simulink model "aero_atc"  (Simulink 6.0)
settings: Solver=ode45  StartTime=0.0  StopTime=60000  MaxStep=.25  RelTol=1e-3
PreLoadFcn:
  | aero_preload_atc
InitFcn:
  | aero_init_atc
values from neighbouring files (symbols this model uses):
  AZ_Sep = get(findobj('Tag','AZ_Sep_edit'),'Value')    [aero_init_atc.m]
  BwPw = get(findobj('Tag','BW_PW_edit'),'Value')    [aero_init_atc.m]
  E = get(findobj('Tag','Antenna_E_edit'),'Value')    [aero_init_atc.m]
  EL_Sep = get(findobj('Tag','EL_Sep_edit'),'Value')    [aero_init_atc.m]
  Lambda = get(findobj('Tag','Wavelength_edit'),'Value')    [aero_init_atc.m]
  Loss = get(findobj('Tag','Losses_edit'),'Value')    [aero_init_atc.m]
  Noise = get(findobj('Tag','Noise_Factor_edit'),'Value')    [aero_init_atc.m]
  Pt = get(findobj('Tag','Trans_Power_edit'),'Value')    [aero_init_atc.m]
  rainfall = get(findobj('Style','radiobutton','Value',[1]),'UserData')    [aero_init_atc.m]
  Rrange = get(findobj('Tag','RADAR_Range_edit'),'Value')    [aero_init_atc.m]
  Rres = get(findobj('Tag','Range_Res_edit'),'Value')    [aero_init_atc.m]
  SNR = get(findobj('Tag','SNR_edit'),'Value')    [aero_init_atc.m]
  Temp = get(findobj('Tag','Working_Temp_edit'),'Value')    [aero_init_atc.m]
libraries: simulink3 x1
CloseFcn:
  | aero_atcscript('close')
settings Model: RequirementInfo=9  CovMetricSettings=d  Creator=The MathWorks Inc.  LastModifiedBy=batserve  ExtModeTrigMode=oneshot  ExtModeArmWhenConnect=off  ExtModeAutoUpdateStatusClock=off
settings DataIOCC: MaxDataPoints=5000  SaveOutput=off  SaveTime=off
settings OptimizationCC: BlockReduction=off  BooleanDataType=off
settings DebuggingCC: CheckExecutionContextPreStartOutputMsg=on  CheckExecutionContextRuntimeOutputMsg=on  SolverPrmCheckMsg=none
settings HardwareCC: TargetUnknown=on

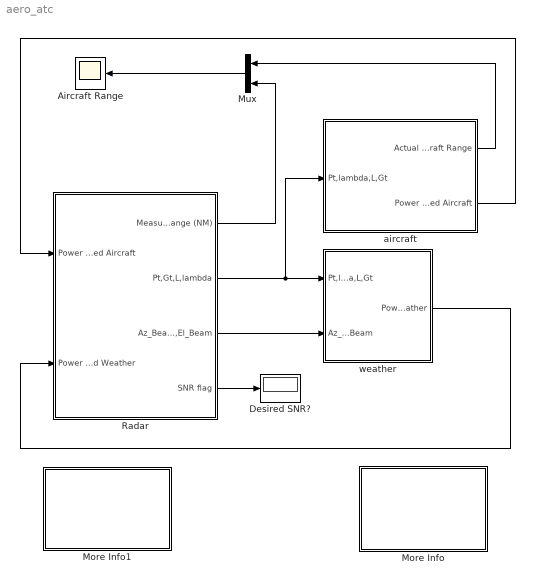
== system aero_atc ==
  Aircraft Range : Scope
      settings: DeleteFcn=simscope BlockIsBeingDestroyed  TimeRange=10300  YMin=0  YMax=65
  Desired SNR? : Display
  More Info : Subsystem  PropExecContextAcrossSSBoundary=on
      settings: OpenFcn=aero_atcscript
      mask Display: disp('Double-click \nhere for \ninformation on \nthis demonstration')
  More Info1 : Subsystem  PropExecContextAcrossSSBoundary=on
      settings: OpenFcn=simcad(bdroot);
      mask Display: disp('Double click\nhere for\nSimulink Help')
  Mux : Mux  Orientation=left  Inputs=2
  Radar : Subsystem  PropExecContextAcrossSSBoundary=on
      mask Display: image(radar)
  aircraft : Subsystem  PropExecContextAcrossSSBoundary=on
      mask Display: image(plane)
  weather : Subsystem  PropExecContextAcrossSSBoundary=on
      mask Display: image(weather);
  wires:
  Radar/2(Pt,Gt,L,lambda) -> aircraft/1(Pt,lambda,L,Gt), weather/1(Pt,lambda,L,Gt)
  Radar/3(Az_Beam,El_Beam) -> weather/2(Az_Beam,El_Beam)
  weather/1(Power Returned Weather) -> Radar/2(Power Received Weather)
  aircraft/2(Power Returned Aircraft) -> Radar/1(Power Received Aircraft)
  Radar/1(Measured Aircraft Range (NM)) -> Mux/2
  aircraft/1(Actual Aircraft Range) -> Mux/1
  Mux/1 -> Aircraft Range/1
  Radar/4(SNR flag) -> Desired SNR?/1

== system aero_atc/More Info ==

== system aero_atc/More Info1 ==

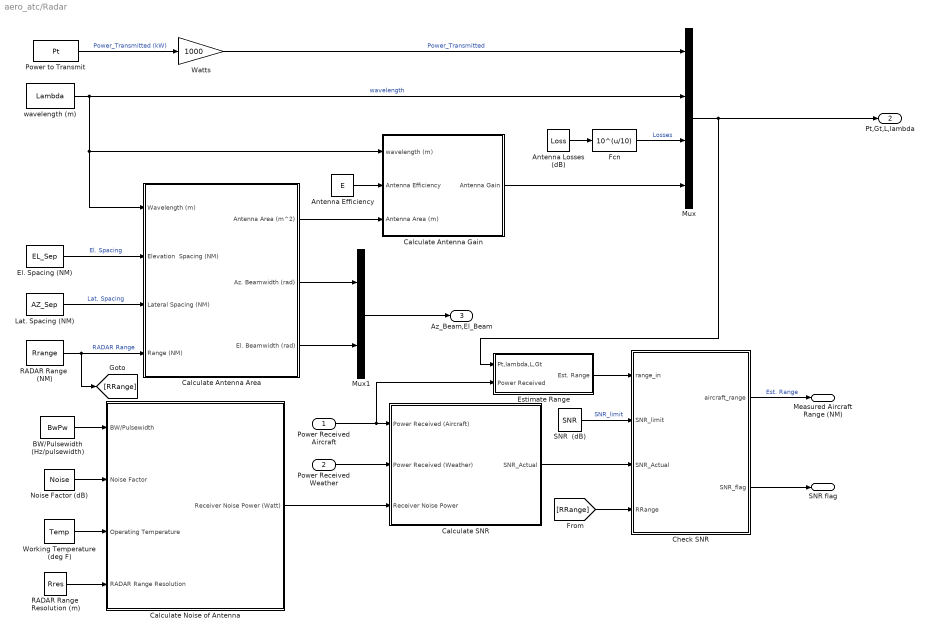
== system aero_atc/Radar ==
  Power Received Aircraft : Inport  Port=1  LatchInput=off
  Power Received Weather : Inport  Port=2  LatchInput=off
  Antenna Efficiency : Constant  Value=E
  Antenna Losses (dB) : Constant  Value=Loss
  BW/Pulsewidth (Hz/pulsewidth) : Constant  Value=BwPw
  Calculate SNR : Subsystem  PropExecContextAcrossSSBoundary=on
  Calculate Antenna Area : Subsystem  PropExecContextAcrossSSBoundary=on
  Calculate Antenna Gain : Subsystem  PropExecContextAcrossSSBoundary=on
  Calculate Noise of Antenna : Subsystem  PropExecContextAcrossSSBoundary=on
  Check SNR : Stateflow chart  PropExecContextAcrossSSBoundary=on
  El. Spacing (NM) : Constant  Value=EL_Sep
  Estimate Range : Subsystem  PropExecContextAcrossSSBoundary=on
  Fcn : Fcn  Expr=10^(u/10)
  Lat. Spacing (NM) : Constant  Value=AZ_Sep
  Mux : Mux
  Mux1 : Mux  Inputs=2
  Noise Factor (dB) : Constant  Value=Noise
  Power to Transmit : Constant  Value=Pt
  RADAR Range  (NM) : Constant  Value=Rrange
  RADAR Range  Resolution (m) : Constant  Value=Rres
  SNR  (dB) : Constant  Value=SNR
  Watts : Gain  Gain=1000  SaturateOnIntegerOverflow=on
  Working Temperature (deg F) : Constant  Value=Temp
  "wavelength (m) " : Constant  Value=Lambda
  Measured Aircraft Range (NM) : Outport
  Pt,Gt,L,lambda : Outport  Port=2
  Az_Beam,El_Beam : Outport  Port=3
  SNR flag : Outport  Port=4
  wires:
  Antenna Efficiency/1 -> Calculate Antenna Gain/2(Antenna Efficiency)
  Lat. Spacing (NM)/1 -> Calculate Antenna Area/3(Lateral Spacing (NM))  "Lat. Spacing"
  El. Spacing (NM)/1 -> Calculate Antenna Area/2(Elevation  Spacing (NM))  "El. Spacing"
  "wavelength (m) "/1 -> Calculate Antenna Area/1(Wavelength (m)), Calculate Antenna Gain/1(wavelength (m)), Mux/2  "wavelength"
  Calculate Antenna Area/1(Antenna Area (m^2)) -> Calculate Antenna Gain/3(Antenna Area (m))
  RADAR Range  (NM)/1 -> Calculate Antenna Area/4(Range (NM)), [RRange]  "RADAR Range"
  RADAR Range  Resolution (m)/1 -> Calculate Noise of Antenna/4(RADAR Range Resolution)
  BW/Pulsewidth (Hz/pulsewidth)/1 -> Calculate Noise of Antenna/1(BW/Pulsewidth)
  Noise Factor (dB)/1 -> Calculate Noise of Antenna/2(Noise Factor)
  Working Temperature (deg F)/1 -> Calculate Noise of Antenna/3(Operating Temperature)
  Calculate Antenna Area/3("El. Beamwidth (rad) ") -> Mux1/2
  Calculate Antenna Area/2("Az. Beamwidth (rad) ") -> Mux1/1
  Mux1/1 -> Az_Beam,El_Beam/1
  Power Received Weather/1 -> Calculate SNR/2(Power Received (Weather))
  Power Received Aircraft/1 -> Calculate SNR/1(Power Received (Aircraft)), Estimate Range/2(Power Received)
  Calculate Noise of Antenna/1(Receiver Noise Power (Watt)) -> Calculate SNR/3(Receiver Noise Power)
  Mux/1 -> Pt,Gt,L,lambda/1, Estimate Range/1(Pt,lambda,L,Gt)
  Calculate Antenna Gain/1("Antenna Gain ") -> Mux/4
  Fcn/1 -> Mux/3  "Losses"
  Watts/1 -> Mux/1  "Power_Transmitted"
  Antenna Losses (dB)/1 -> Fcn/1
  Power to Transmit/1 -> Watts/1  "Power_Transmitted (kW)"
  Check SNR/1(aircraft_range) -> Measured Aircraft Range (NM)/1  "Est. Range"
  Estimate Range/1(Est. Range) -> Check SNR/1(range_in)
  SNR  (dB)/1 -> Check SNR/2(SNR_limit)  "SNR_limit"
  Calculate SNR/1(SNR_Actual) -> Check SNR/3(SNR_Actual)
  [RRange] -> Check SNR/4(RRange)
  Check SNR/2(SNR_flag) -> SNR flag/1

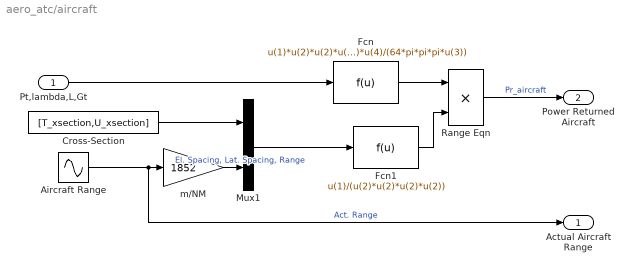
== system aero_atc/aircraft ==
  Pt,lambda,L,Gt : Inport  Port=1  LatchInput=off
  Aircraft Range : Sin  Amplitude=25  Bias=35  Frequency=0.0025  SampleTime=0
  Cross-Section : FromWorkspace  VariableName=[T_xsection,U_xsection]  SampleTime=0  Interpolate=off  OutputAfterFinalValue=Holding final value
  Fcn : Fcn  Expr=u(1)*u(2)*u(2)*u(4)*u(4)/(64*pi*pi*pi*u(3))
  Fcn1 : Fcn  Expr=u(1)/(u(2)*u(2)*u(2)*u(2))
  Mux1 : Mux  Inputs=2
  Range Eqn : Product  SaturateOnIntegerOverflow=on  RndMeth=Zero  InputSameDT=on
  m/NM : Gain  Gain=1852  SaturateOnIntegerOverflow=on
  Actual Aircraft Range : Outport
  Power Returned Aircraft : Outport  Port=2
  wires:
  Pt,lambda,L,Gt/1 -> Fcn/1
  Cross-Section/1 -> Mux1/1
  Mux1/1 -> Fcn1/1
  m/NM/1 -> Mux1/2  "El. Spacing, Lat. Spacing, Range"
  Fcn/1 -> Range Eqn/1
  Range Eqn/1 -> Power Returned Aircraft/1  "Pr_aircraft"
  Fcn1/1 -> Range Eqn/2
  Aircraft Range/1 -> Actual Aircraft Range/1, m/NM/1  "Act. Range"

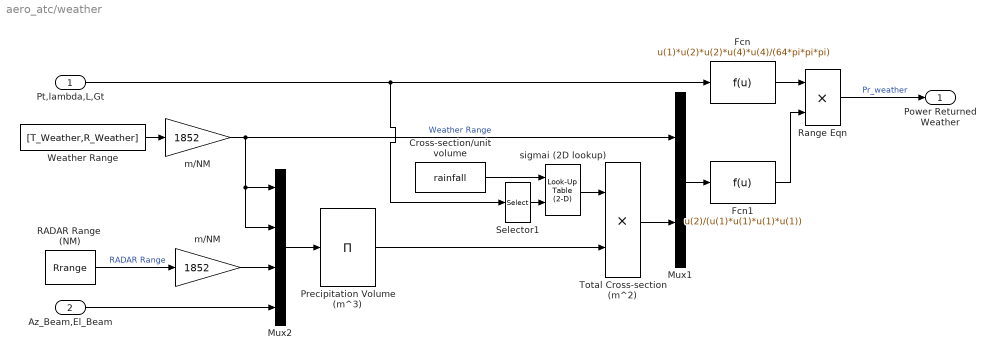
== system aero_atc/weather ==
  Pt,lambda,L,Gt : Inport  Port=1  LatchInput=off
  Az_Beam,El_Beam : Inport  Port=2  LatchInput=off
  Cross-section/unit volume : Constant  Value=rainfall
  Fcn : Fcn  Expr=u(1)*u(2)*u(2)*u(4)*u(4)/(64*pi*pi*pi)
  Fcn1 : Fcn  Expr=u(2)/(u(1)*u(1)*u(1)*u(1))
  Mux1 : Mux  Inputs=2
  Mux2 : Mux
  Precipitation Volume (m^3) : Product  Inputs=*  SaturateOnIntegerOverflow=on  RndMeth=Zero  InputSameDT=on
  RADAR Range  (NM) : Constant  Value=Rrange
  Range Eqn : Product  SaturateOnIntegerOverflow=on  RndMeth=Zero  InputSameDT=on
  Selector1 : Selector  Elements=2  InputPortWidth=4
  Total Cross-section (m^2) : Product  SaturateOnIntegerOverflow=on  RndMeth=Zero  InputSameDT=on
  Weather Range : FromWorkspace  VariableName=[T_Weather,R_Weather]  SampleTime=0  Interpolate=off  OutputAfterFinalValue=Holding final value
  m/NM : Gain  Gain=1852  SaturateOnIntegerOverflow=on
  "m/NM " : Gain  Gain=1852  SaturateOnIntegerOverflow=on
  sigmai (2D lookup) : simulink3/Functions & Tables/Look-Up Table (2-D)  x=rainfall_bp  y=lambda_bp  t=sigma_table
  Power Returned Weather : Outport
  wires:
  Mux2/1 -> Precipitation Volume (m^3)/1
  m/NM/1 -> Mux2/3
  RADAR Range  (NM)/1 -> m/NM/1  "RADAR Range"
  Az_Beam,El_Beam/1 -> Mux2/4
  "m/NM "/1 -> Mux1/1, Mux2/1, Mux2/2  "Weather Range"
  Mux1/1 -> Fcn1/1
  Weather Range/1 -> "m/NM "/1
  sigmai (2D lookup)/1 -> Total Cross-section (m^2)/1
  Pt,lambda,L,Gt/1 -> Selector1/1, Fcn/1
  Precipitation Volume (m^3)/1 -> Total Cross-section (m^2)/2
  Fcn1/1 -> Range Eqn/2
  Selector1/1 -> sigmai (2D lookup)/2
  Cross-section/unit volume/1 -> sigmai (2D lookup)/1
  Total Cross-section (m^2)/1 -> Mux1/2
  Fcn/1 -> Range Eqn/1
  Range Eqn/1 -> Power Returned Weather/1  "Pr_weather"

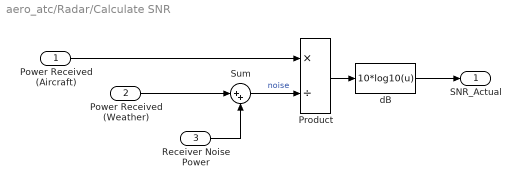
== system aero_atc/Radar/Calculate SNR ==
  Power Received (Aircraft) : Inport  Port=1  LatchInput=off
  Power Received (Weather) : Inport  Port=2  LatchInput=off
  Receiver Noise Power : Inport  Port=3  LatchInput=off
  Product : Product  Inputs=*/  SaturateOnIntegerOverflow=on  RndMeth=Zero  InputSameDT=on
  Sum : Sum  Inputs=|++  SaturateOnIntegerOverflow=on  InputSameDT=on
  dB : Fcn  Expr=10*log10(u)
  SNR_Actual : Outport
  wires:
  Sum/1 -> Product/2  "noise"
  Power Received (Aircraft)/1 -> Product/1
  Power Received (Weather)/1 -> Sum/1
  Receiver Noise Power/1 -> Sum/2
  Product/1 -> dB/1
  dB/1 -> SNR_Actual/1

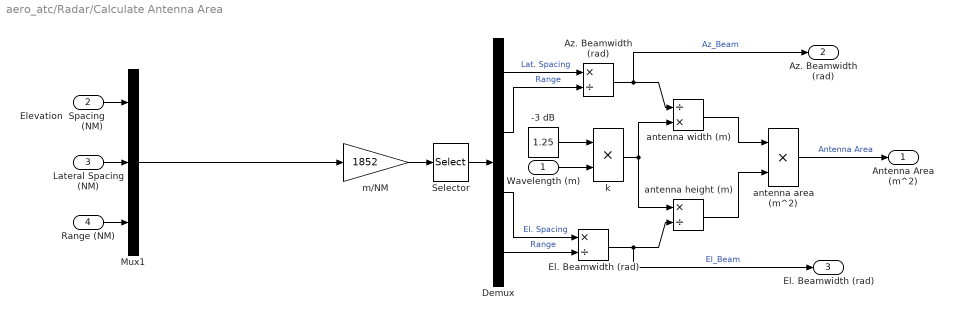
== system aero_atc/Radar/Calculate Antenna Area ==
  Wavelength (m) : Inport  Port=1  LatchInput=off
  Elevation  Spacing (NM) : Inport  Port=2  LatchInput=off
  Lateral Spacing (NM) : Inport  Port=3  LatchInput=off
  Range (NM) : Inport  Port=4  LatchInput=off
  "-3 dB  " : Constant  Value=1.25
  Az. Beamwidth (rad) : Product  Inputs=*/  SaturateOnIntegerOverflow=on  RndMeth=Zero  InputSameDT=on
  Demux : Demux
  El. Beamwidth (rad) : Product  Inputs=*/  SaturateOnIntegerOverflow=on  RndMeth=Zero  InputSameDT=on
  Mux1 : Mux  Inputs=3
  Selector : Selector  Elements=[1 3 2 3]  InputPortWidth=3
  antenna area (m^2) : Product  SaturateOnIntegerOverflow=on  RndMeth=Zero  InputSameDT=on
  antenna height (m) : Product  Inputs=*/  SaturateOnIntegerOverflow=on  RndMeth=Zero  InputSameDT=on
  antenna width (m) : Product  Inputs=/*  SaturateOnIntegerOverflow=on  RndMeth=Zero  InputSameDT=on
  k : Product  Inputs=**  SaturateOnIntegerOverflow=on  RndMeth=Zero  InputSameDT=on
  m/NM : Gain  Gain=1852  SaturateOnIntegerOverflow=on
  Antenna Area (m^2) : Outport
  "Az. Beamwidth (rad) " : Outport  Port=2
  "El. Beamwidth (rad) " : Outport  Port=3
  wires:
  m/NM/1 -> Selector/1
  Selector/1 -> Demux/1
  Demux/1 -> Az. Beamwidth (rad)/1  "Lat. Spacing"
  Demux/2 -> Az. Beamwidth (rad)/2  "Range"
  Demux/3 -> El. Beamwidth (rad)/1  "El. Spacing"
  Demux/4 -> El. Beamwidth (rad)/2  "Range"
  Wavelength (m)/1 -> k/2
  "-3 dB  "/1 -> k/1
  k/1 -> antenna height (m)/1, antenna width (m)/2
  Az. Beamwidth (rad)/1 -> antenna width (m)/1, "Az. Beamwidth (rad) "/1  "Az_Beam"
  antenna width (m)/1 -> antenna area (m^2)/1
  antenna height (m)/1 -> antenna area (m^2)/2
  antenna area (m^2)/1 -> Antenna Area (m^2)/1  "Antenna Area"
  El. Beamwidth (rad)/1 -> antenna height (m)/2, "El. Beamwidth (rad) "/1  "El_Beam"
  Mux1/1 -> m/NM/1
  Elevation  Spacing (NM)/1 -> Mux1/1
  Lateral Spacing (NM)/1 -> Mux1/2
  Range (NM)/1 -> Mux1/3

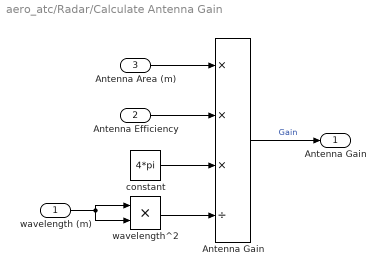
== system aero_atc/Radar/Calculate Antenna Gain ==
  wavelength (m) : Inport  Port=1  LatchInput=off
  Antenna Efficiency : Inport  Port=2  LatchInput=off
  Antenna Area (m) : Inport  Port=3  LatchInput=off
  Antenna Gain : Product  Inputs=***/  SaturateOnIntegerOverflow=on  RndMeth=Zero  InputSameDT=on
  constant : Constant  Value=4*pi
  wavelength^2 : Product  SaturateOnIntegerOverflow=on  RndMeth=Zero  InputSameDT=on
  "Antenna Gain " : Outport
  wires:
  Antenna Efficiency/1 -> Antenna Gain/2
  constant/1 -> Antenna Gain/3
  wavelength^2/1 -> Antenna Gain/4
  Antenna Area (m)/1 -> Antenna Gain/1
  Antenna Gain/1 -> "Antenna Gain "/1  "Gain"
  wavelength (m)/1 -> wavelength^2/2, wavelength^2/1

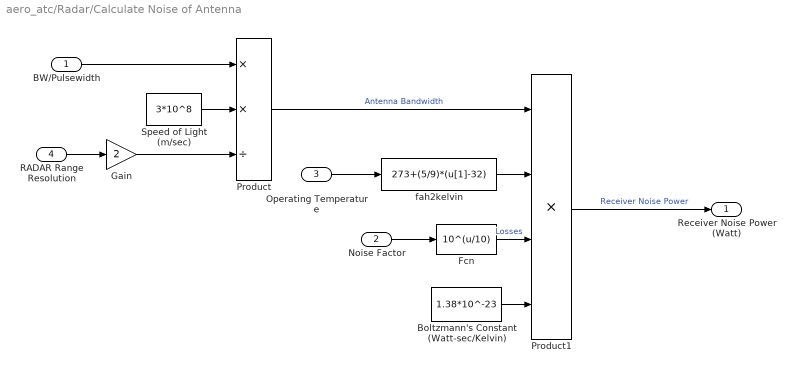
== system aero_atc/Radar/Calculate Noise of Antenna ==
  BW/Pulsewidth : Inport  Port=1  LatchInput=off
  Noise Factor : Inport  Port=2  LatchInput=off
  Operating Temperature : Inport  Port=3  LatchInput=off
  RADAR Range Resolution : Inport  Port=4  LatchInput=off
  Boltzmann's Constant (Watt-sec/Kelvin) : Constant  Value=1.38*10^-23
  Fcn : Fcn  Expr=10^(u/10)
  Gain : Gain  Gain=2  SaturateOnIntegerOverflow=on
  Product : Product  Inputs=**/  SaturateOnIntegerOverflow=on  RndMeth=Zero  InputSameDT=on
  Product1 : Product  Inputs=4  SaturateOnIntegerOverflow=on  RndMeth=Zero  InputSameDT=on
  Speed of Light (m/sec) : Constant  Value=3*10^8
  fah2kelvin : Fcn  Expr=273+(5/9)*(u[1]-32)
  Receiver Noise Power (Watt) : Outport
  wires:
  Speed of Light (m/sec)/1 -> Product/2
  Gain/1 -> Product/3
  BW/Pulsewidth/1 -> Product/1
  RADAR Range Resolution/1 -> Gain/1
  Product/1 -> Product1/1  "Antenna Bandwidth"
  fah2kelvin/1 -> Product1/2
  Boltzmann's Constant (Watt-sec/Kelvin)/1 -> Product1/4
  Product1/1 -> Receiver Noise Power (Watt)/1  "Receiver Noise Power"
  Noise Factor/1 -> Fcn/1
  Fcn/1 -> Product1/3  "Losses"
  Operating Temperature/1 -> fah2kelvin/1

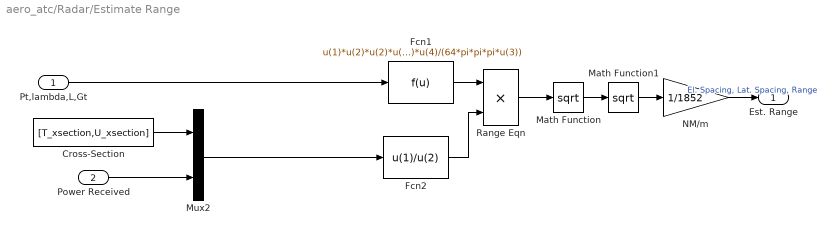
== system aero_atc/Radar/Estimate Range ==
  Pt,lambda,L,Gt : Inport  Port=1  LatchInput=off
  Power Received : Inport  Port=2  LatchInput=off
  Cross-Section : FromWorkspace  VariableName=[T_xsection,U_xsection]  SampleTime=0
  Fcn1 : Fcn  Expr=u(1)*u(2)*u(2)*u(4)*u(4)/(64*pi*pi*pi*u(3))
  Fcn2 : Fcn  Expr=u(1)/u(2)
  Math Function : Math  Operator=sqrt  SaturateOnIntegerOverflow=on
  Math Function1 : Math  Operator=sqrt  SaturateOnIntegerOverflow=on
  Mux2 : Mux  Inputs=2
  NM/m : Gain  Gain=1/1852  SaturateOnIntegerOverflow=on
  Range Eqn : Product  SaturateOnIntegerOverflow=on  RndMeth=Zero  InputSameDT=on
  Est. Range : Outport
  wires:
  Pt,lambda,L,Gt/1 -> Fcn1/1
  Fcn1/1 -> Range Eqn/1
  Fcn2/1 -> Range Eqn/2
  Range Eqn/1 -> Math Function/1
  Math Function/1 -> Math Function1/1
  Math Function1/1 -> NM/m/1
  NM/m/1 -> Est. Range/1  "El. Spacing, Lat. Spacing, Range"
  Cross-Section/1 -> Mux2/1
  Power Received/1 -> Mux2/2
  Mux2/1 -> Fcn2/1

== stateflow chart Radar/Check SNR ==
  settings: updateMethod=CONTINUOUS
  state Visability [parallel]
    state detect
      during: aircraft_range = range_in;
    state no_detect
      during: aircraft_range =0;
    (default) -> (junction 9)
    (junction 9) -> no_detect : [(SNR_Actual <= 6) || (range_in > RRange)]
        | { aircraft_range =0;}
    (junction 9) -> detect : [(SNR_Actual > 6) && (range_in <= RRange) ]
        | { aircraft_range = range_in;}
    no_detect -> detect : [(SNR_Actual > 6) && (range_in <= RRange)]
        | { aircraft_range = range_in;}
    detect -> no_detect : [(SNR_Actual <= 6) || (range_in > RRange)]
        | { aircraft_range = 0;}
  state SNR [parallel]
    state Less_than
    state Equal_to_or_Greater_than
    (default) -> (junction 10)
    (junction 10) -> Less_than : [SNR_Actual < SNR_limit]{SNR_flag = 0;}
    (junction 10) -> Equal_to_or_Greater_than : [SNR_Actual >= SNR_limit]{SNR_flag = 1;}
    Less_than -> Equal_to_or_Greater_than : [SNR_Actual >= SNR_limit]{SNR_flag = 1;}
    Equal_to_or_Greater_than -> Less_than : [SNR_Actual < SNR_limit]{SNR_flag = 0;}
  data: range_in input double size=1; SNR_limit input double size=1; SNR_Actual input double size=1; aircraft_range output double size=1 =0; RRange input double size=1; SNR_flag output double size=1
